simulink model "sim_MPC_Heli_int_du_2017a"  (R2017a)
settings: Solver=ode4  StartTime=0.0  StopTime=inf  FixedStep=0.01  RelTol=1e-3
InitFcn:
  | run('initialize_system_du.m')
values from neighbouring files (symbols this model uses):
  Ac = At    [initialize_system_du.m]
  Ad = ds.a    [initialize_system.m]    (also in initialize_system_du.m)
  Bc = Bt    [initialize_system_du.m]
  Bd = ds.b    [initialize_system.m]    (also in initialize_system_du.m)
  Cc = Ct    [initialize_system_du.m]
  Cd = ds.c    [initialize_system.m]    (also in initialize_system_du.m)
  th_op = -10*pi/180    (= -0.174532925199)    [initialize_system.m]    (also in initialize_system_du.m)
  Vmp_op = (Kyy*m_heli*g*cos(th_op)*l_cm) / (Kyy*Kpp - Kyp*Kpy)    [initialize_system.m]    (also in initialize_system_du.m)
  Vmy_op = (Kyp*Vmp_op) / (Kyy)    [initialize_system.m]    (also in initialize_system_du.m)
  xt_op = [th_op;yw_op;w_th_op;w_yw_op;0;0]    [initialize_system_du.m]
  yw_op = pi/2    (= 1.57079632679)    [initialize_system.m]    (also in initialize_system_du.m)
undefined symbols (not defined in the file or in its folder): L
libraries: simulink_extras x2, realtime_pacer_lib x1
settings Model: Creator=engen  LastModifiedBy=eirik.engen
settings DataIOCC: ReturnWorkspaceOutputs=on
settings SFSimCC: SimUseLocalCustomCode=on
settings RTWCC: RTWUseLocalCustomCode=on

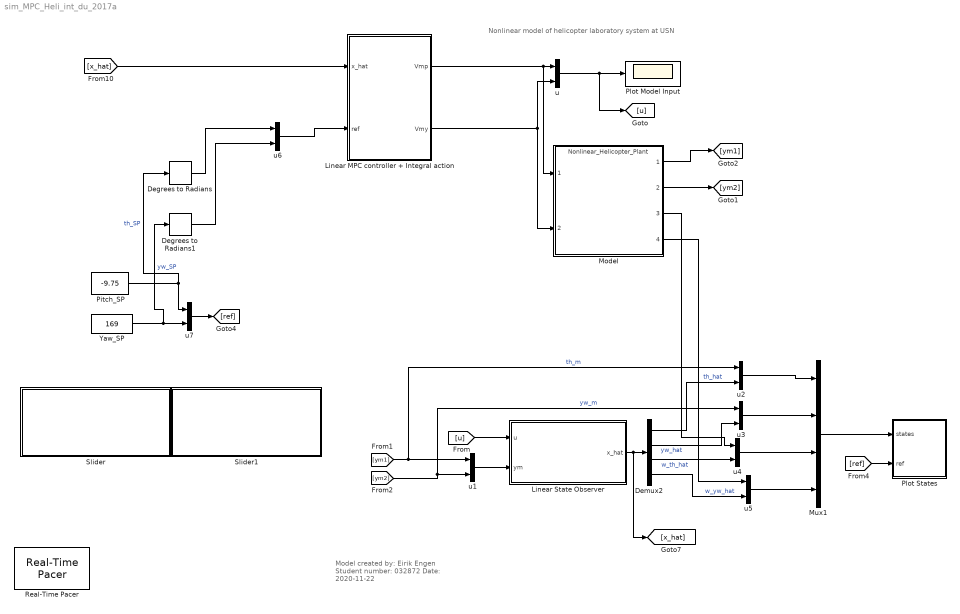
== system sim_MPC_Heli_int_du_2017a ==
  note: Model created by: Eirik Engen
      | Student number: 032872
      | Date: 2020-11-22
  note: Nonlinear model of helicopter laboratory system at USN
  Degrees to Radians : simulink_extras/Transformations/Degrees to Radians
  Degrees to Radians1 : simulink_extras/Transformations/Degrees to Radians
  Demux2 : Demux
  Linear MPC controller + Integral action : Subsystem
  Linear State Observer : Subsystem
  Model : ModelReference  ModelNameDialog=Nonlinear_Helicopter_Plant.slxp  ModelReferenceVersion=1.53  CopyOfModelProtected=on
  Mux1 : Mux
  Pitch_SP : Constant  Value=-9.75  SampleTime=-1
  Plot Model Input : Scope
  Plot States : Subsystem
  Real-Time Pacer : realtime_pacer_lib/Real-Time Pacer  simTimePerRealTime=1
  Slider : Subsystem  DialogController=hmiCreateDDGDialog  IsWebBlock=on  mask(MWDashboardBlock){webBlockId=17649b03-82fe-4141-b83e-204aa1d8152d, webBlockType=slider, ShowInLibBrowser=on, ShowInitialText=on, HMISrcModelName=sim_MPC_Heli_int_du_2017a}
      mask prompts: webBlockId "WebBlock Id"; webBlockType "WebBlock Type"; HMISrcModelName "Source Model"
      mask help: Set value to tune parameters or variables.
      mask Help: helpview([docroot '/mapfiles/simulink.map'], 'hmi_slider')
      mask Display:
      | if strcmp(get_param(bdroot(gcb),'BlockDiagramType'),'library')
      |  image([(matlabroot) '/toolbox/simulink/hmi/icons/Slider.png'])
      | end
  Slider1 : Subsystem  DialogController=hmiCreateDDGDialog  IsWebBlock=on  mask(MWDashboardBlock){webBlockId=393126f9-46b9-4254-924b-546b90f379c0, webBlockType=slider, ShowInLibBrowser=on, ShowInitialText=on, HMISrcModelName=sim_MPC_Heli_int_du_2017a}
      mask prompts: webBlockId "WebBlock Id"; webBlockType "WebBlock Type"; HMISrcModelName "Source Model"
      mask help: Set value to tune parameters or variables.
      mask Help: helpview([docroot '/mapfiles/simulink.map'], 'hmi_slider')
      mask Display:
      | if strcmp(get_param(bdroot(gcb),'BlockDiagramType'),'library')
      |  image([(matlabroot) '/toolbox/simulink/hmi/icons/Slider.png'])
      | end
  Yaw_SP : Constant  Value=169  SampleTime=-1
  u{,1..7} (8 alike) : Mux  Inputs=2
  wires:
  Model/1 -> [ym1]
  Model/2 -> [ym2]
  Model/3 -> u4/1
  Model/4 -> u5/1
  u/1 -> [u], Plot Model Input/1
  [u] -> Linear State Observer/1(u)
  u1/1 -> Linear State Observer/2(ym)
  Linear State Observer/1(x_hat) -> [x_hat], Demux2/1
  Mux1/1 -> Plot States/1(states)
  u2/1 -> Mux1/1
  u3/1 -> Mux1/2
  Demux2/1 -> u2/2  "th_hat"
  Demux2/2 -> u3/2  "yw_hat"
  u5/1 -> Mux1/4
  u4/1 -> Mux1/3
  [ym1] -> u2/1, u1/1  "th_m"
  Demux2/4 -> u5/2  "w_yw_hat"
  Demux2/3 -> u4/2  "w_th_hat"
  [ym2] -> u3/1, u1/2  "yw_m"
  Pitch_SP/1 -> u7/1, Degrees to Radians/1  "th_SP"
  Yaw_SP/1 -> Degrees to Radians1/1, u7/2  "yw_SP"
  Degrees to Radians/1 -> u6/1
  Degrees to Radians1/1 -> u6/2
  u7/1 -> [ref]
  [ref] -> Plot States/2(ref)
  Linear MPC controller + Integral action/2(Vmy) -> Model/2, u/2
  Linear MPC controller + Integral action/1(Vmp) -> Model/1, u/1
  [x_hat] -> Linear MPC controller + Integral action/1(x_hat)
  u6/1 -> Linear MPC controller + Integral action/2(ref)

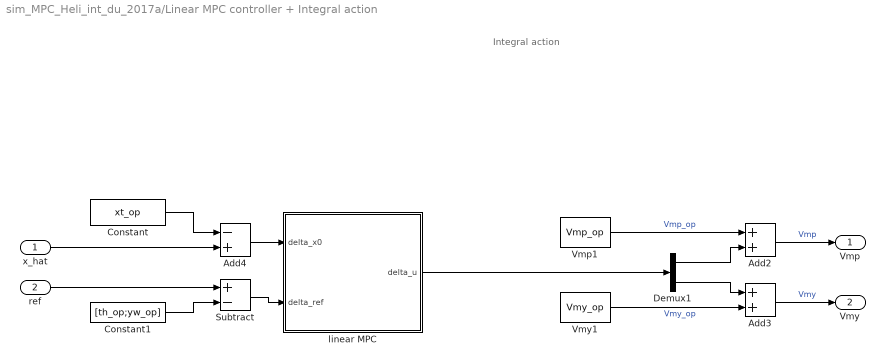
== system sim_MPC_Heli_int_du_2017a/Linear MPC controller + Integral action ==
  note: Integral action
  x_hat : Inport
  ref : Inport  Port=2
  Add2 : Sum  OutMin=0  OutMax=3
  Add3 : Sum  OutMin=0  OutMax=3
  Add4 : Sum  Inputs=-+
  Constant : Constant  Value=xt_op
  Constant1 : Constant  Value=[th_op;yw_op]
  Demux1 : Demux  Outputs=2
  Subtract : Sum  Inputs=+-
  Vmp1 : Constant  Value=Vmp_op  SampleTime=-1
  Vmy1 : Constant  Value=Vmy_op  SampleTime=-1
  linear MPC : Subsystem
  Vmp : Outport
  Vmy : Outport  Port=2
  wires:
  Subtract/1 -> linear MPC/2(delta_ref)
  Vmp1/1 -> Add2/1  "Vmp_op"
  linear MPC/1(delta_u) -> Demux1/1
  Add2/1 -> Vmp/1  "Vmp"
  Add3/1 -> Vmy/1  "Vmy"
  Add4/1 -> linear MPC/1(delta_x0)
  Constant/1 -> Add4/1
  Demux1/2 -> Add3/1
  ref/1 -> Subtract/1
  x_hat/1 -> Add4/2
  Constant1/1 -> Subtract/2
  Demux1/1 -> Add2/2
  Vmy1/1 -> Add3/2  "Vmy_op"

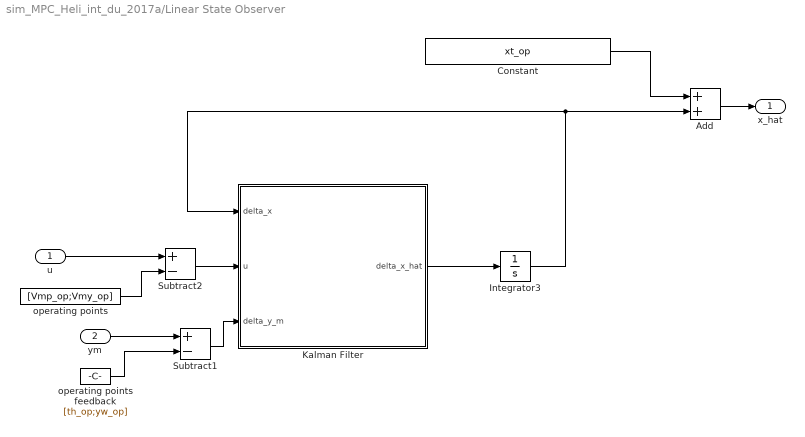
== system sim_MPC_Heli_int_du_2017a/Linear State Observer ==
  u : Inport
  ym : Inport  Port=2
  Add : Sum
  Constant : Constant  Value=xt_op
  Integrator3 : Integrator
  Kalman Filter : MATLAB Function  TreatAsAtomicUnit=on
  Subtract1 : Sum  Inputs=+-
  Subtract2 : Sum  Inputs=+-
  operating points : Constant  Value=[Vmp_op;Vmy_op]
  operating points feedback : Constant  Value=[th_op;yw_op]
  x_hat : Outport
  wires:
  Kalman Filter/1(delta_x_hat) -> Integrator3/1
  Integrator3/1 -> Kalman Filter/1(delta_x), Add/2
  Subtract1/1 -> Kalman Filter/3(delta_y_m)
  ym/1 -> Subtract1/1
  operating points feedback/1 -> Subtract1/2
  Add/1 -> x_hat/1
  Subtract2/1 -> Kalman Filter/2(u)
  u/1 -> Subtract2/1
  operating points/1 -> Subtract2/2
  Constant/1 -> Add/1

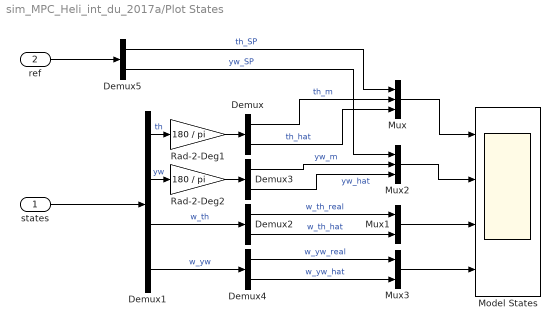
== system sim_MPC_Heli_int_du_2017a/Plot States ==
  states : Inport
  ref : Inport  Port=2
  Demux{,2..5} (5 alike) : Demux  Outputs=2
  Demux1 : Demux
  Model States : Scope  NumInputPorts=4
  Mux : Mux  Inputs=3
  Mux1 : Mux  Inputs=2
  Mux2 : Mux  Inputs=3
  Mux3 : Mux  Inputs=2
  Rad-2-Deg1 : Gain  Gain=180 / pi
  Rad-2-Deg2 : Gain  Gain=180 / pi
  wires:
  states/1 -> Demux1/1
  Demux/1 -> Mux/2  "th_m"
  Demux/2 -> Mux/3  "th_hat"
  Demux3/1 -> Mux2/2  "yw_m"
  Demux3/2 -> Mux2/3  "yw_hat"
  Demux2/1 -> Mux1/1  "w_th_real"
  Demux2/2 -> Mux1/2  "w_th_hat"
  Demux4/1 -> Mux3/1  "w_yw_real"
  Demux4/2 -> Mux3/2  "w_yw_hat"
  Demux1/1 -> Rad-2-Deg1/1  "th"
  Demux1/2 -> Rad-2-Deg2/1  "yw"
  Demux1/3 -> Demux2/1  "w_th"
  Demux1/4 -> Demux4/1  "w_yw"
  Mux/1 -> Model States/1
  Mux2/1 -> Model States/2
  Mux1/1 -> Model States/3
  Mux3/1 -> Model States/4
  ref/1 -> Demux5/1
  Demux5/2 -> Mux2/1  "yw_SP"
  Demux5/1 -> Mux/1  "th_SP"
  Rad-2-Deg1/1 -> Demux/1
  Rad-2-Deg2/1 -> Demux3/1

== system sim_MPC_Heli_int_du_2017a/Slider ==

== system sim_MPC_Heli_int_du_2017a/Slider1 ==

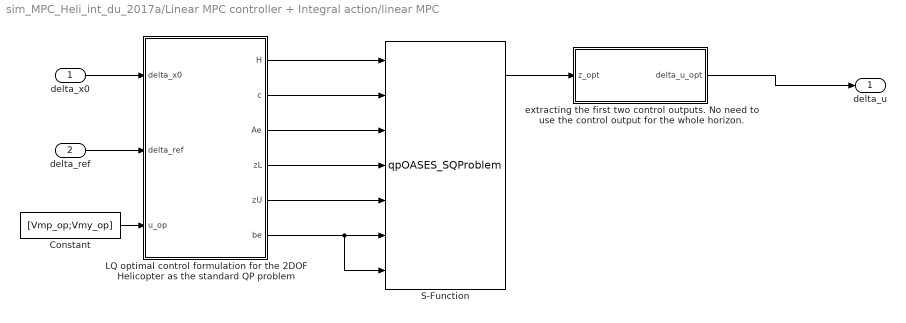
== system sim_MPC_Heli_int_du_2017a/Linear MPC controller + Integral action/linear MPC ==
  delta_x0 : Inport
  delta_ref : Inport  Port=2
  Constant : Constant  Value=[Vmp_op;Vmy_op]
  LQ optimal control formulation for the 2DOF Helicopter as the standard QP problem : MATLAB Function  TreatAsAtomicUnit=on
  S-Function : S-Function  FunctionName=qpOASES_SQProblem  SFunctionDeploymentMode=off  EnableBusSupport=off
  extracting the first two control outputs. No need to use the control output for the whole horizon. : MATLAB Function  TreatAsAtomicUnit=on
  delta_u : Outport
  wires:
  delta_x0/1 -> LQ optimal control formulation for the 2DOF Helicopter as the standard QP problem/1(delta_x0)
  delta_ref/1 -> LQ optimal control formulation for the 2DOF Helicopter as the standard QP problem/2(delta_ref)
  LQ optimal control formulation for the 2DOF Helicopter as the standard QP problem/1(H) -> S-Function/1
  LQ optimal control formulation for the 2DOF Helicopter as the standard QP problem/2(c) -> S-Function/2
  LQ optimal control formulation for the 2DOF Helicopter as the standard QP problem/3(Ae) -> S-Function/3
  LQ optimal control formulation for the 2DOF Helicopter as the standard QP problem/4(zL) -> S-Function/4
  LQ optimal control formulation for the 2DOF Helicopter as the standard QP problem/5(zU) -> S-Function/5
  LQ optimal control formulation for the 2DOF Helicopter as the standard QP problem/6(be) -> S-Function/7, S-Function/6
  S-Function/1 -> extracting the first two control outputs. No need to use the control output for the whole horizon./1(z_opt)
  Constant/1 -> LQ optimal control formulation for the 2DOF Helicopter as the standard QP problem/3(u_op)
  extracting the first two control outputs. No need to use the control output for the whole horizon./1(delta_u_opt) -> delta_u/1

== matlab function sim_MPC_Heli_int_du_2017a/Linear State Observer/Kalman Filter ==
  data: delta_x input; u input; delta_x_hat output size=6; delta_y_m input; Ac parameter; Bc parameter; Cc parameter; L parameter
function delta_x_hat = linear_state_observer(delta_x, u,delta_y_m,Ac,Bc,Cc,L)
    %apriori state
    delta_x_hat = Ac*delta_x + Bc*u;
    %estimated output    
    y_hat = Cc*delta_x;
    % aposteriori state
    delta_x_hat = delta_x_hat + L*(delta_y_m - y_hat);

== matlab function sim_MPC_Heli_int_du_2017a/Linear MPC controller + Integral action/linear MPC/LQ optimal control formulation for the 2DOF Helicopter as the standard QP problem ==
  data: delta_x0 input; H output; delta_ref input; u_op input; c output; Ae output; zL output; zU output; be output; Ad parameter; Bd parameter; Cd parameter
function [H,c,Ae,zL,zU,be] = QP_formulation_Heli(delta_x0,delta_ref, u_op, Ad, Bd, Cd)
    % System matrices of discrete time model is pre-loaded in Simulink and 
    % Ad, Bd and Cd matrices are configured as parameters in this function.
    %
    % Configuration
    N = 12; % prediction horizon length
    %weighting matrices
    Q=diag([1 1]); %tuning weight for error: there are 2 (size(ny))
    P=diag([1e-3 1e-3]);            %tuning weight for inputs: there are 2 (size(nu))
     %size of state-matrix, output-matrix and input-matrix
    nx = size(Ad,1); nu = size(Bd,2); ny = size(Cd,1);
    %size of the unknow vector z
    nz = N*(nx + nu + 2*ny);
    % Define boundaries
    uL = 0*ones(nu,1) - u_op; 
    uU = 3*ones(nu,1) - u_op;
    xL = -inf*ones(nx,1);
    xU = inf*ones(nx,1);
    eL = -inf*ones(ny,1);
    eU = inf*ones(ny,1);
    yL = -inf*ones(ny,1);
    yU = inf*ones(ny,1);
    
    
    %initial values of the states
    x0 = delta_x0;
    
    % Define reference for the whole prediction/simulation length
    % row # 1: pitch angle
    % row # 2: yaw angle
    r = [ones(1,N).*delta_ref(1);                 
         ones(1,N).*delta_ref(2)];    
    
    % build matrices
    H11 = kron(eye(N),P); 
    H22 = zeros(N*nx,N*nx); 
    H33 = kron(eye(N),Q);
    H44 = zeros(N*ny,N*ny);
    H_mat = blkdiag(H11,H22,H33,H44);
    %reshape to vector form to support qpOASES
    H = H_mat(:);
    c = zeros(nz,1);
    %constraints (from process model)
    % State equation reference
    Ae1u = -kron(eye(N),Bd);
    Ae1x = eye(N*nx)-kron(diag(ones(N-abs(-1),1),-1),Ad); 
    Ae1e = zeros(N*nx,N*ny); % eq 1 is states, hence nx rows, and errors are ny cols.
    Ae1y = zeros(N*nx,N*ny);
    be1 = [Ad*x0;zeros((N-1)*nx,1)];
    %Measurement equation reference
    Ae2u = zeros(N*ny,N*nu); % eq 2 is measurement eq, ny cols, nu inputs
    Ae2x = -kron(eye(N),Cd); 
    Ae2e = zeros(N*ny,N*ny); 
    Ae2y = eye(N*ny);
    be2 = zeros(N*ny,1);
    %Error equation reference
    Ae3u = zeros(N*ny,N*nu); % eq 3 is error, ny lines, and nu inputs
    Ae3x = zeros(N*ny,N*nx); 
    Ae3e = eye(N*ny);
    Ae3y = eye(N*ny);
    % reshape r for be3
    be3 = reshape(r,N*ny,1);
    % Define final Ae matrix
    Ae_mat=[Ae1u Ae1x Ae1e Ae1y 
            Ae2u Ae2x Ae2e Ae2y 
            Ae3u Ae3x Ae3e Ae3y];
    %reshape to vector form to support qpOASES
    Ae = Ae_mat(:);
    % Define final be vector
    be=[be1;be2;be3];
    %bounds
    zL=[kron(ones(N,1),uL)
        kron(ones(N,1),xL)
        kron(ones(N,1),eL)
        kron(ones(N,1),yL)]; 
    
    zU=[kron(ones(N,1),uU)
        kron(ones(N,1),xU)
        kron(ones(N,1),eU)
        kron(ones(N,1),yU)];

== matlab function sim_MPC_Heli_int_du_2017a/Linear MPC controller + Integral action/linear MPC/extracting the first two control outputs. No need to use the control output for the whole horizon. ==
  data: z_opt input; delta_u_opt output
function delta_u_opt = extract_first_control(z_opt)

delta_u_opt = z_opt(1:2);
